simulink model "Lab2_Sim_Int"  (R2019a)
settings: Solver=VariableStepAuto  StartTime=0.0  StopTime=0.4  RelTol=1e-3
values from neighbouring files (symbols this model uses):
  a =     [calculatedFunctions.mat]    (also in computeLinearization.m = L_f_h - b*u)
  b =     [calculatedFunctions.mat]    (also in computeLinearization.m = diff(L_f_h, u))
  diffeo =     [calculatedFunctions.mat]
  F = FInt(1 : 4)    [Lab2.m]
  H = FInt(5)    [Lab2.m]
settings Model: Creator=DELL  LastModifiedBy=Ricardo Wang

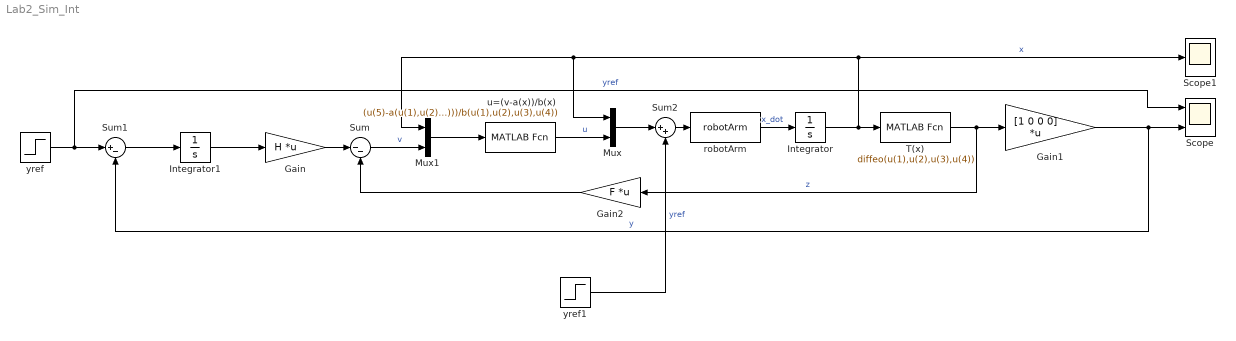
== system Lab2_Sim_Int ==
  Gain : Gain  Gain=H  Multiplication=Matrix(K*u) (u vector)
  Gain1 : Gain  Gain=[1 0 0 0]  Multiplication=Matrix(K*u) (u vector)
  Gain2 : Gain  Gain=F  Multiplication=Matrix(K*u) (u vector)
  Integrator : Integrator
  Integrator1 : Integrator
  Mux : Mux  Inputs=2
  Mux1 : Mux  Inputs=2
  Scope : Scope  NumInputPorts=2
  Scope1 : Scope
  Sum : Sum  Inputs=|--
  Sum1 : Sum  Inputs=|+-
  Sum2 : Sum  Inputs=|++
  T(x) : MATLABFcn  MATLABFcn=diffeo(u(1),u(2),u(3),u(4))  OutputDimensions=4
  robotArm : MATLABFcn  MATLABFcn=robotArm  OutputDimensions=4
  u=(v-a(x))/b(x) : MATLABFcn  MATLABFcn=(u(5)-a(u(1),u(2),u(3),u(4)))/b(u(1),u(2),u(3),u(4))  OutputDimensions=1
  yref : Step  Time=0  After=0  SampleTime=0
  yref1 : Step  Time=0.2  After=0.5  SampleTime=0
  wires:
  u=(v-a(x))/b(x)/1 -> Mux/2  "u"
  Gain1/1 -> Scope/2, Sum1/2  "y"
  T(x)/1 -> Gain2/1, Gain1/1  "z"
  Gain/1 -> Sum/1
  Mux1/1 -> u=(v-a(x))/b(x)/1
  Sum/1 -> Mux1/2  "v"
  yref/1 -> Scope/1, Sum1/1  "yref"
  Gain2/1 -> Sum/2
  Integrator/1 -> T(x)/1, Scope1/1, Mux/1, Mux1/1  "x"
  robotArm/1 -> Integrator/1  "x_dot"
  Sum1/1 -> Integrator1/1
  Integrator1/1 -> Gain/1
  Mux/1 -> Sum2/1
  Sum2/1 -> robotArm/1
  yref1/1 -> Sum2/2  "yref"
